simulink model "two_leader_formation"  (R2019a)
settings: Solver=VariableStepAuto  StartTime=0.0  StopTime=10.0  RelTol=1e-3
undefined symbols (not defined in the file): B, I, L
settings Model: Creator=DELL  LastModifiedBy=DELL

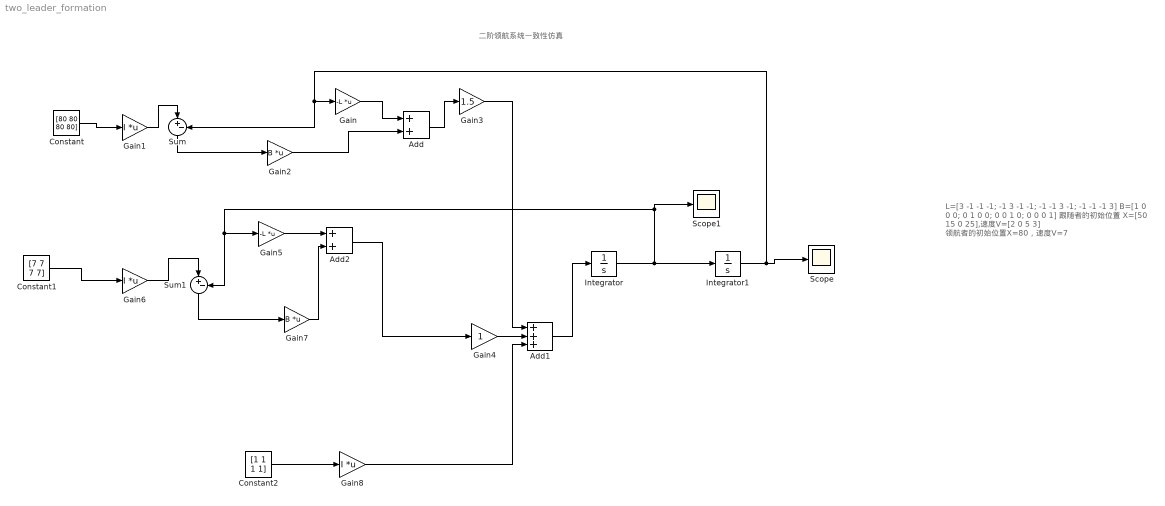
== system two_leader_formation ==
  note: 二阶领航系统一致性仿真
  note: L=[3 -1 -1 -1;
      | -1 3 -1 -1;
      | -1 -1 3 -1;
      | -1 -1 -1 3]
      |
      | B=[1 0 0 0;
      | 0 1 0 0;
      | 0 0 1 0;
      | 0 0 0 1]
      |
      | 跟随者的初始位置 X=[50 15 0 25],速度V=[2 0 5 3]
      | 领航者的初始位置X=80，速度V=7
  Add : Sum
  Add1 : Sum  Inputs=+++
  Add2 : Sum
  Constant : Constant  Value=[80 80 80 80]
  Constant1 : Constant  Value=[7 7 7 7]
  Constant2 : Constant  Value=[1 1 1 1]
  Gain : Gain  Gain=-L  Multiplication=Matrix(K*u)
  Gain1 : Gain  Gain=I  Multiplication=Matrix(K*u)
  Gain2 : Gain  Gain=B  Multiplication=Matrix(K*u)
  Gain3 : Gain  Gain=1.5
  Gain4 : Gain
  Gain5 : Gain  Gain=-L  Multiplication=Matrix(K*u)
  Gain6 : Gain  Gain=I  Multiplication=Matrix(K*u)
  Gain7 : Gain  Gain=B  Multiplication=Matrix(K*u)
  Gain8 : Gain  Gain=I  Multiplication=Matrix(K*u)
  Integrator : Integrator  InitialCondition=[2 0 5 3]
  Integrator1 : Integrator  InitialCondition=[50 15 0 25]
  Scope : Scope
  Scope1 : Scope
  Sum : Sum  Inputs=|+-
  Sum1 : Sum  Inputs=|+-
  wires:
  Integrator/1 -> Scope1/1, Sum1/2, Gain5/1, Integrator1/1
  Integrator1/1 -> Sum/2, Gain/1, Scope/1
  Constant/1 -> Gain1/1
  Gain1/1 -> Sum/1
  Sum/1 -> Gain2/1
  Gain/1 -> Add/1
  Gain2/1 -> Add/2
  Add/1 -> Gain3/1
  Add1/1 -> Integrator/1
  Gain3/1 -> Add1/1
  Gain4/1 -> Add1/2
  Constant1/1 -> Gain6/1
  Gain6/1 -> Sum1/1
  Sum1/1 -> Gain7/1
  Gain5/1 -> Add2/1
  Gain7/1 -> Add2/2
  Add2/1 -> Gain4/1
  Constant2/1 -> Gain8/1
  Gain8/1 -> Add1/3
